simulink model "p2nftool_simulink"  (Simulink 7.7)
settings: Solver=ode45  StartTime=0.0  StopTime=10.0  RelTol=1e-3
libraries: neural x17
(part 1 of 3)
settings Model: Creator=Aditya  LastModifiedBy=Aditya

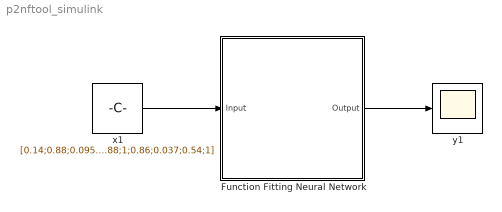
== system p2nftool_simulink ==
  Function Fitting Neural Network : Subsystem
      mask Description: Function Fitting Neural Network
      mask Display: e = 0.06;c1 = [120 150 230]/255;c2 = ([120 150 230]+0)/383;c3 = ([120 150 230]+128)/383;patch([0 1 1 0],[0 0 1 1],c1);patch([0 1 1 1-e 1-e 0+e],[0 0 1 1-e 0+e 0+e],c2);patch([0 0 1 1-e 0+e 0+e],[0 1 1 1-e 1-e 0+e],c3);plot([0 1 1 0 0],[0 0 1 1 0]);fprintf('NNET');port_label('input',1,' Input');port_label('output',1,'Output ');
  x1 : Constant  Value=[0.14;0.88;0.095;0.35;0.59;0.59;0.67;0.65;0.43;0.14;0.75;0.24;0.65;0.86;0.084;0.97;0.031;0.84;0.84;0.05;0.55;0.94;0.32;0.81;0.6;0.79;0.8;0.05;0.28;0.65;0.49;0.97;0.75;0.57;0.3;0.26;0.89;0.45;0.82;0.098;0.86;0.028;0.9;0.9;0.52;0.12;0.18;0.71;0.83;0.035;0.76;0.96;0.34;0.64;0.34;0.22;0.79;0.72;0.28;0.58;0.42;0.092;0.024;0.49;0.28;0.34;0.29;0.17;0.4;0.7;0.2;0.67;0.44;0.43;0.18;0.19;0.62;0.27;0.56;0.94;0.71;0.68;0.96;0.78;0.61;0.95;0.06;0.27;0.99;0.77;0.48;0.68;0.42;0.38;0.21;0.38;0.03;0.47;0.33;0.98;0.56;0.85;0.41;0.46;0.83;0.99;0.52;0.93;0.74;0.57;0.97;0.82;0.96;0.65;0.38;0.48;0.91;0.015;0.16;0.47;0.54;0.06;0.66;0.89;0.11;0.44;0.28;0.99;0.61;0.25;0.13;0.55;0.83;0.84;0.83;0.2;0.54;0.87;0.12;0.86;0.9;0.22;0.077;0.47;0.84;0.47;0.41;0.5;0.13;0.13;0.87;0.6;0.27;0.86;0.058;0.46;0.72;0.34;0.4;0.53;0.89;0.78;0.069;0.28;0.38;0.86;0.42;0.24;0.6;0.48;0.9;0.93;0.82;0.71;0.74;0.9;0.065;0.34;0.0043;0.83;0.51;0.37;0.23;0.53;0.29;0.068;0.085;0.068;0.41;0.12;0.44;0.9;0.35;0.12;0.57;0.88;0.35;0.042;0.14;0.077;0.74;0.46;0.67;0.7;0.57;0.63;0.88;0.66;0.88;0.47;0.14;0.068;0.71;0.31;0.67;0.65;0.53;0.72;0.5;0.49;0.5;0.94;0.39;0.12;0.24;0.68;0.84;0.97;0.22;0.76;0.58;0.4;0.51;0.5;0.65;0.74;0.3;0.09;0.83;0.39;0.78;0.18;0.11;0.91;0.88;1;0.86;0.037;0.54;1]  SampleTime=1
      mask Display: e = 0.06;c1 = [120 230 180]/255;c2 = ([120 230 180]+0)/(256+128);c3 = ([120 230 180]+128)/(256+128);patch([0 1 1 0],[0 0 1 1],c1);patch([0 1 1 1-e 1-e 0+e],[0 0 1 1-e 0+e 0+e],c2);patch([0 0 1 1-e 0+e 0+e],[0 1 1 1-e 1-e 0+e],c3);plot([0 1 1 0 0],[0 0 1 1 0]);disp('Constant');
  y1 : Scope
      settings: DataFormat=Array
      mask Display: e = 0.06;c1 = [120 230 180]/255;c2 = ([120 230 180]+0)/(256+128);c3 = ([120 230 180]+128)/(256+128);patch([0 1 1 0],[0 0 1 1],c1);patch([0 1 1 1-e 1-e 0+e],[0 0 1 1-e 0+e 0+e],c2);patch([0 0 1 1-e 0+e 0+e],[0 1 1 1-e 1-e 0+e],c3);plot([0 1 1 0 0],[0 0 1 1 0]);plot([0.15 0.85 0.85 0.15 0.15],[0.5 0.5 0.85 0.85 0.5]);
  wires:
  x1/1 -> Function Fitting Neural Network/1(Input)
  Function Fitting Neural Network/1(Output) -> y1/1

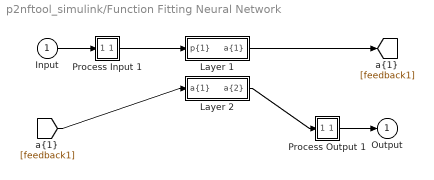
== system p2nftool_simulink/Function Fitting Neural Network ==
  Input : Inport  PortDimensions=250
      mask Display: e = 0.06;c1 = [120 230 180]/255;c2 = ([120 230 180]+0)/(256+128);c3 = ([120 230 180]+128)/(256+128);patch([0 1 1 0],[0 0 1 1],c1);patch([0 1 1 1-e 1-e 0+e],[0 0 1 1-e 0+e 0+e],c2);patch([0 0 1 1-e 0+e 0+e],[0 1 1 1-e 1-e 0+e],c3);plot([0 1 1 0 0],[0 0 1 1 0]);
  Layer 1 : Subsystem
      mask Display: e = 0.06;c1 = [120 150 230]/255;c2 = ([120 150 230]+0)/383;c3 = ([120 150 230]+128)/383;patch([0 1 1 0],[0 0 1 1],c1);patch([0 1 1 1-e 1-e 0+e],[0 0 1 1-e 0+e 0+e],c2);patch([0 0 1 1-e 0+e 0+e],[0 1 1 1-e 1-e 0+e],c3);plot([0 1 1 0 0],[0 0 1 1 0]);
  Layer 2 : Subsystem
      mask Display: e = 0.06;c1 = [120 150 230]/255;c2 = ([120 150 230]+0)/383;c3 = ([120 150 230]+128)/383;patch([0 1 1 0],[0 0 1 1],c1);patch([0 1 1 1-e 1-e 0+e],[0 0 1 1-e 0+e 0+e],c2);patch([0 0 1 1-e 0+e 0+e],[0 1 1 1-e 1-e 0+e],c3);plot([0 1 1 0 0],[0 0 1 1 0]);
  Process Input 1 : Subsystem
      mask Display: e = 0.06;c1 = [120 150 230]/255;c2 = ([120 150 230]+0)/383;c3 = ([120 150 230]+128)/383;patch([0 1 1 0],[0 0 1 1],c1);patch([0 1 1 1-e 1-e 0+e],[0 0 1 1-e 0+e 0+e],c2);patch([0 0 1 1-e 0+e 0+e],[0 1 1 1-e 1-e 0+e],c3);plot([0 1 1 0 0],[0 0 1 1 0]);
  Process Output 1 : Subsystem
      mask Display: e = 0.06;c1 = [120 150 230]/255;c2 = ([120 150 230]+0)/383;c3 = ([120 150 230]+128)/383;patch([0 1 1 0],[0 0 1 1],c1);patch([0 1 1 1-e 1-e 0+e],[0 0 1 1-e 0+e 0+e],c2);patch([0 0 1 1-e 0+e 0+e],[0 1 1 1-e 1-e 0+e],c3);plot([0 1 1 0 0],[0 0 1 1 0]);
  Output : Outport  InitialOutput=0
      mask Display: e = 0.06;c1 = [120 230 180]/255;c2 = ([120 230 180]+0)/(256+128);c3 = ([120 230 180]+128)/(256+128);patch([0 1 1 0],[0 0 1 1],c1);patch([0 1 1 1-e 1-e 0+e],[0 0 1 1-e 0+e 0+e],c2);patch([0 0 1 1-e 0+e 0+e],[0 1 1 1-e 1-e 0+e],c3);plot([0 1 1 0 0],[0 0 1 1 0]);
  wires:
  Input/1 -> Process Input 1/1(x)
  Process Output 1/1(y) -> Output/1
  Process Input 1/1(p) -> Layer 1/1("p{1}")
  Layer 1/1("a{1}") -> [feedback1]
  [feedback1] -> Layer 2/1("a{1} ")
  Layer 2/1("a{2}") -> Process Output 1/1(a)

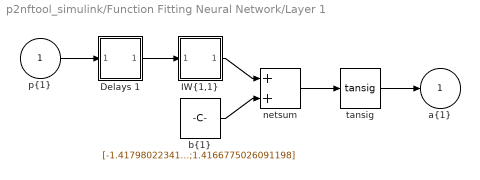
== system p2nftool_simulink/Function Fitting Neural Network/Layer 1 ==
  "p{1}" : Inport  PortDimensions=247
      mask Display: e = 0.06;c1 = [120 230 180]/255;c2 = ([120 230 180]+0)/(256+128);c3 = ([120 230 180]+128)/(256+128);patch([0 1 1 0],[0 0 1 1],c1);patch([0 1 1 1-e 1-e 0+e],[0 0 1 1-e 0+e 0+e],c2);patch([0 0 1 1-e 0+e 0+e],[0 1 1 1-e 1-e 0+e],c3);plot([0 1 1 0 0],[0 0 1 1 0]);
  Delays 1 : Subsystem
      mask Display: e = 0.06;c1 = [120 150 230]/255;c2 = ([120 150 230]+0)/383;c3 = ([120 150 230]+128)/383;patch([0 1 1 0],[0 0 1 1],c1);patch([0 1 1 1-e 1-e 0+e],[0 0 1 1-e 0+e 0+e],c2);patch([0 0 1 1-e 0+e 0+e],[0 1 1 1-e 1-e 0+e],c3);plot([0 1 1 0 0],[0 0 1 1 0]);disp('0');
  "IW{1,1}" : Subsystem
      mask Display: e = 0.06;c1 = [120 150 230]/255;c2 = ([120 150 230]+0)/383;c3 = ([120 150 230]+128)/383;patch([0 1 1 0],[0 0 1 1],c1);patch([0 1 1 1-e 1-e 0+e],[0 0 1 1-e 0+e 0+e],c2);patch([0 0 1 1-e 0+e 0+e],[0 1 1 1-e 1-e 0+e],c3);plot([0 1 1 0 0],[0 0 1 1 0]);disp('W');
  "b{1}" : Constant  Value=[-1.4179802234186696;-1.09460213536941;0.81514063966848649;-0.49229912761746891;-0.1249783039630278;-0.2000150392778885;-0.46243985430235329;0.78624382911976132;1.1056778923148194;1.4166775026091198]
      mask Display: e = 0.06;c1 = [120 150 230]/255;c2 = ([120 150 230]+0)/383;c3 = ([120 150 230]+128)/383;patch([0 1 1 0],[0 0 1 1],c1);patch([0 1 1 1-e 1-e 0+e],[0 0 1 1-e 0+e 0+e],c2);patch([0 0 1 1-e 0+e 0+e],[0 1 1 1-e 1-e 0+e],c3);plot([0 1 1 0 0],[0 0 1 1 0]);disp('b');
  netsum : Sum  Inputs=2  SaturateOnIntegerOverflow=on  InputSameDT=on  OutDataTypeStr=Inherit: Same as first input
      mask Display: e = 0.06;c1 = [120 150 230]/255;c2 = ([120 150 230]+0)/383;c3 = ([120 150 230]+128)/383;patch([0 1 1 0],[0 0 1 1],c1);patch([0 1 1 1-e 1-e 0+e],[0 0 1 1-e 0+e 0+e],c2);patch([0 0 1 1-e 0+e 0+e],[0 1 1 1-e 1-e 0+e],c3);plot([0 1 1 0 0],[0 0 1 1 0]);disp('+');
  tansig : neural/Transfer Functions/tansig  SystemSampleTime=-1
  "a{1}" : Outport  InitialOutput=[0;0;0;0;0;0;0;0;0;0]
      mask Display: e = 0.06;c1 = [120 230 180]/255;c2 = ([120 230 180]+0)/(256+128);c3 = ([120 230 180]+128)/(256+128);patch([0 1 1 0],[0 0 1 1],c1);patch([0 1 1 1-e 1-e 0+e],[0 0 1 1-e 0+e 0+e],c2);patch([0 0 1 1-e 0+e 0+e],[0 1 1 1-e 1-e 0+e],c3);plot([0 1 1 0 0],[0 0 1 1 0]);
  wires:
  "p{1}"/1 -> Delays 1/1("p{1}")
  Delays 1/1("pd{1,1}") -> "IW{1,1}"/1("pd{1,1}")
  "IW{1,1}"/1("iz{1,1}") -> netsum/1
  "b{1}"/1 -> netsum/2
  netsum/1 -> tansig/1
  tansig/1 -> "a{1}"/1

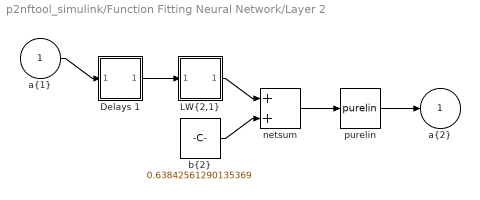
== system p2nftool_simulink/Function Fitting Neural Network/Layer 2 ==
  "a{1} " : Inport  PortDimensions=10
      mask Display: e = 0.06;c1 = [120 230 180]/255;c2 = ([120 230 180]+0)/(256+128);c3 = ([120 230 180]+128)/(256+128);patch([0 1 1 0],[0 0 1 1],c1);patch([0 1 1 1-e 1-e 0+e],[0 0 1 1-e 0+e 0+e],c2);patch([0 0 1 1-e 0+e 0+e],[0 1 1 1-e 1-e 0+e],c3);plot([0 1 1 0 0],[0 0 1 1 0]);
  Delays 1 : Subsystem
      mask Display: e = 0.06;c1 = [120 150 230]/255;c2 = ([120 150 230]+0)/383;c3 = ([120 150 230]+128)/383;patch([0 1 1 0],[0 0 1 1],c1);patch([0 1 1 1-e 1-e 0+e],[0 0 1 1-e 0+e 0+e],c2);patch([0 0 1 1-e 0+e 0+e],[0 1 1 1-e 1-e 0+e],c3);plot([0 1 1 0 0],[0 0 1 1 0]);disp('0');
  "LW{2,1}" : Subsystem
      mask Display: e = 0.06;c1 = [120 150 230]/255;c2 = ([120 150 230]+0)/383;c3 = ([120 150 230]+128)/383;patch([0 1 1 0],[0 0 1 1],c1);patch([0 1 1 1-e 1-e 0+e],[0 0 1 1-e 0+e 0+e],c2);patch([0 0 1 1-e 0+e 0+e],[0 1 1 1-e 1-e 0+e],c3);plot([0 1 1 0 0],[0 0 1 1 0]);disp('W');
  "b{2}" : Constant  Value=0.63842561290135369
      mask Display: e = 0.06;c1 = [120 150 230]/255;c2 = ([120 150 230]+0)/383;c3 = ([120 150 230]+128)/383;patch([0 1 1 0],[0 0 1 1],c1);patch([0 1 1 1-e 1-e 0+e],[0 0 1 1-e 0+e 0+e],c2);patch([0 0 1 1-e 0+e 0+e],[0 1 1 1-e 1-e 0+e],c3);plot([0 1 1 0 0],[0 0 1 1 0]);disp('b');
  netsum : Sum  Inputs=2  SaturateOnIntegerOverflow=on  InputSameDT=on  OutDataTypeStr=Inherit: Same as first input
      mask Display: e = 0.06;c1 = [120 150 230]/255;c2 = ([120 150 230]+0)/383;c3 = ([120 150 230]+128)/383;patch([0 1 1 0],[0 0 1 1],c1);patch([0 1 1 1-e 1-e 0+e],[0 0 1 1-e 0+e 0+e],c2);patch([0 0 1 1-e 0+e 0+e],[0 1 1 1-e 1-e 0+e],c3);plot([0 1 1 0 0],[0 0 1 1 0]);disp('+');
  purelin : neural/Transfer Functions/purelin  SystemSampleTime=-1
  "a{2}" : Outport  InitialOutput=0
      mask Display: e = 0.06;c1 = [120 230 180]/255;c2 = ([120 230 180]+0)/(256+128);c3 = ([120 230 180]+128)/(256+128);patch([0 1 1 0],[0 0 1 1],c1);patch([0 1 1 1-e 1-e 0+e],[0 0 1 1-e 0+e 0+e],c2);patch([0 0 1 1-e 0+e 0+e],[0 1 1 1-e 1-e 0+e],c3);plot([0 1 1 0 0],[0 0 1 1 0]);
  wires:
  "a{1} "/1 -> Delays 1/1("p{2}")
  Delays 1/1("pd{2,1}") -> "LW{2,1}"/1("ad{2,1}")
  "LW{2,1}"/1("lz{2,1}") -> netsum/1
  "b{2}"/1 -> netsum/2
  netsum/1 -> purelin/1
  purelin/1 -> "a{2}"/1

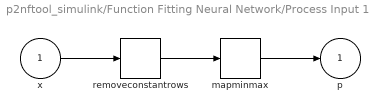
== system p2nftool_simulink/Function Fitting Neural Network/Process Input 1 ==
  x : Inport  PortDimensions=250
      mask Display: e = 0.06;c1 = [120 230 180]/255;c2 = ([120 230 180]+0)/(256+128);c3 = ([120 230 180]+128)/(256+128);patch([0 1 1 0],[0 0 1 1],c1);patch([0 1 1 1-e 1-e 0+e],[0 0 1 1-e 0+e 0+e],c2);patch([0 0 1 1-e 0+e 0+e],[0 1 1 1-e 1-e 0+e],c3);plot([0 1 1 0 0],[0 0 1 1 0]);
  mapminmax : neural/Processing Functions/mapminmax  SystemSampleTime=-1  xmin=[0.28314095380123011;0.0014657625514411762;1.1970013108086204e-053;0;3.1940747747761186e-136;1.0738088237835023e-008;0.057013843843753034;0.60598157151527954;0.97115785079355899;0.23505552379416098;0.0015659409791624098;1.7067224722511445e-053;0;8.0368942823302572e-061;4.5103371866006794e-009;0.04123819331054894;0.47948358616284426;0.88558703437196162;0.21511995153872421;0.0010808819751517852;2.8250692334704583e-046;2.4009309165522609e-100;2.9707490367076884e-027;9.6683230662484232e-007;0.022724192555573834;0.3373513142068964;0.94606039580726742;0.83381807044158585;0.21660287739295905;0.00088853633165548963;1.7009716611458678e-033;6.6780336252168211e-038;5.0696194701202741e-008;0.0036192264717555211;0.041362148979468445;0.30981136666700104;0.59801786498896425;0.79746531298425982;0.22315144476727924;0.0021495963375243315;8.1846160068553859e-025;2.8239914066742661e-017;0.0031408384351054031;0.042889224861903372;0.16276386773841925;0.40408038951216474;0.29066305341648024;0.76797757181136939;0.22877389647410262;0.0044456023366028895;5.600834653331497e-018;4.9394259822708177e-005;0.036840087959434539;0.17965949427207609;0.32363552339254342;0.45835299547326352;0.094130813464933724;0.75302798590493225;0.23743798347569076;0.0069561268877913604;6.4536346515668317e-010;0.008381002087497539;0.15708349906195013;0.30441724262311659;0.36780124819343157;0.2185871738005285;0.016765306036066845;0.74823061163344928;0.23947729804432752;0.010714512873083724;0.0010541317728196189;0.06157188394951027;0.28625369595068767;0.34844665670906477;0.28103818782833434;0.058728583468080235;0.0010252578856185749;0.74321854178214442;0.23689947649479201;0.018726205322830435;0.01403763154106394;0.22602305913201878;0.33322483120237623;0.33385806818767932;0.089161720319027582;0.0074641188499559637;4.9961895725867701e-014;0.73482943796744249;0.25372073679541962;0.029679290835118714;0.088110073989501325;0.30087532130095329;0.32980140896340393;0.16333410471453411;0.017268639637258193;2.1255584492753245e-005;3.393723053715393e-030;0.71603300903271727;0.28086288081641786;0.070765696337695222;0.25962114262595792;0.29530395857824981;0.29469508150713242;0.042775243878743575;0.0029717096345041856;2.9208044705741375e-016;6.5528308610418704e-056;0.69175545649373782;0.29982802434084543;0.20379814240139515;0.27454377432499888;0.27997276525054976;0.12616229517130753;0.0096590827511273004;1.3644328135045095e-006;2.142759325296534e-030;4.040485592604963e-142;0.66009817247140257;0.32061678791653081;0.2682547532557979;0.27174385900521508;0.20641766013384005;0.037985710799232193;0.0013807033350987767;1.3012635462117102e-015;5.4320946234375216e-057;1.7591464959013825e-240;0.6172769879756197;0.34847790967374298;0.26501955306395414;0.24801128848847065;0.060440114839899084;0.0055485797080829314;1.7011821839009803e-005;1.267314796215441e-026;4.0942538416128276e-118;0;0.55298588875176991;0.39441141595760654;0.24783748213069953;0.11231138884518392;0.010163982524210212;0.00014263917490065886;8.4779138948903329e-012;4.2832420373506433e-043;1.3914284431877022e-183;0;0.44408275342157744;0.45739136644383088;0.21373527300401277;0.030371879562093255;0.00095751904960731358;1.5885247614363501e-006;6.148043824133868e-020;7.3970467026419826e-081;1.4934597127927122e-257;0;0.26243962974132995;0.48079214069904203;0.26231548541471439;0.036602136267184941;0.00060628096867560799;1.2785305836116123e-008;1.1751484874139984e-028;1.1824443720758194e-113;1.5841675491774084e-254;0;0.090633848716506302;0.34771902491284706;0.38815621070205064;0.074059197286721362;0.003659510261993704;1.2345059166718358e-008;8.313897839456496e-019;4.7510923797345716e-037;4.5302986409558723e-159;0;0.010447510961658907;0.12022109545632396;0.43641885135063363;0.17835412356961261;0.023094869323530314;0.0036055987469813863;1.6562419958457672e-006;2.3336559312165858e-018;1.2249443391194443e-049;7.8777061358525906e-305;2.9236537014494795e-005;0.012406243347218964;0.14829252040733829;0.46412790611608706;0.26210222673708705 ...(+1093 chars)]  xmax=[0.54696499822519751;0.018097615199448878;1.1211625874404843e-008;5.6770535681185055e-031;3.0020232501492485e-023;0.0021391516298108959;0.14989077001407924;1;1;0.51285806504859077;0.012524359149825833;3.7565294910936581e-008;8.8658980841575836e-016;8.8232922508452755e-016;0.001431874497486966;0.11011541950728011;0.74534542491818523;1;0.48923990729976458;0.010269229460599905;0.00012832810780790373;2.2351799345579169e-007;1.1761696155131968e-007;0.0079013681222223249;0.17244731798578716;0.71244774902097929;1;1;0.48140245816606869;0.047806463657213097;0.0081972329787444211;0.00086126759741684059;0.00067631735814793108;0.054522031032458694;0.44327965809411135;0.92459203478062935;1;1;0.49019971138734014;0.17395100080588385;0.065005975793286361;0.01416422714286911;0.012751094148073646;0.20944713469156914;0.78827123663686649;0.87081878078898467;0.95513016761074909;1;0.51122174001432474;0.29403679313756742;0.18568212819115559;0.075803332242896079;0.078401394267904906;0.50135204144083989;0.9664167423402531;0.58456418046873104;0.91739553578710931;1;0.53971323573207386;0.29149662177536673;0.27410880384568065;0.1837507683046567;0.29524394301616924;0.84674198186133631;0.84210071990954583;0.42497663820874571;0.88784360430489151;1;0.57121324179208999;0.22637434602283085;0.28034774373112925;0.26868308271974917;0.59953438584907626;0.97047208655755235;0.50805015525697472;0.34234261762679447;0.87771026590275036;1;0.60074874094814346;0.1916976426070201;0.25414704427969675;0.44993057603357373;0.88913380145795928;0.78092906980325061;0.25708018546662409;0.30771110138826629;0.87022341791434699;1;0.617306656443951;0.19934536258060637;0.3230232905928398;0.68829336578133204;0.95490583236234927;0.43227229211606583;0.22921735464334314;0.29281982938187762;0.85988787364640351;1;0.60630227597781849;0.30945921967509815;0.57138434730137322;0.91429431990444288;0.71818200551782518;0.26394601892423619;0.21426386186227164;0.28369191206670286;0.84562505813256228;1;0.56823312027864892;0.44863329749984288;0.71906026058361971;0.92350828111072714;0.3747432970237301;0.22909478028122401;0.19935616204016754;0.27379410767962531;0.8266315756856335;1;0.51953034271202558;0.60295589781616798;0.91300857377332856;0.66280494491038633;0.22143189882557401;0.2026398062267977;0.1962579230845605;0.31999660638663485;0.80287348923773216;1;0.59296613606001092;0.68686554535086453;0.87309352639261761;0.38035071945566451;0.19048604266347183;0.17957438027237879;0.19276008856692992;0.37383438414826858;0.77561353621643292;1;0.66370203949103279;0.81071578487663132;0.63855594243678315;0.18363161767842476;0.16886869838772173;0.16759119141941323;0.22916253663769068;0.41022006167831676;0.75522032032662323;1;0.73729449658897717;0.7538058199151334;0.3771078802273462;0.15562663623401607;0.15415334753614637;0.16006433070656098;0.29132092095713402;0.43491866548201041;0.75875179823799987;1;0.77180671800562406;0.5668273239134819;0.17155060451941492;0.1329185837986466;0.14311963764645053;0.15322599053717373;0.37231070306965769;0.45173063997351182;0.75898683140048251;0.83129415315023303;0.78769388341964497;0.6903898422838507;0.44895919763123077;0.1310799125816258;0.13227596328915173;0.20184463272049286;0.4103151322505435;0.46903573008910326;0.75524943678441836;0.54304909791427902;0.78030741474702103;0.79441543065435416;0.71400559919879147;0.41985876969231978;0.12847278188546379;0.27306427097241653;0.42596678627353968;0.47506640461712185;0.74784590697831133;0.15994733323285074;0.51367456324893335;0.76588478994661346;0.79540230108298482;0.74664876613427333;0.39156046661972882;0.34114884070619123;0.45291405207552665;0.48456629233600629;0.73631043009063002;0.00022893929550700675;0.11306261647576715;0.42301243689598156;0.73475156560803945;0.78957771166163848;0.76512552649234056;0.38458568107385055;0.47257093304093056;0.47483300931247441;0.71685442986576109;1.3818041240619991e-008;0.00074138417223213555;0.065984006680153626;0.31244947587072502;0.6524693757289467;0.77720367695162929;0.77128579804533637 ...(+697 chars)]  ymin=-1  ymax=1
  removeconstantrows : neural/Processing Functions/removeconstantrows  SystemSampleTime=-1  inputSize=250  keep=[2 3 4 5 6 7 8 9 11 12 13 14 15 16 17 18 19 21 22 23 24 25 26 27 28 29 30 31 32 33 34 35 36 37 38 39 40 41 42 43 44 45 46 47 48 49 50 51 52 53 54 55 56 57 58 59 60 61 62 63 64 65 66 67 68 69 70 71 72 73 74 75 76 77 78 79 80 81 82 83 84 85 86 87 88 89 90 91 92 93 94 95 96 97 98 99 100 101 102 103 104 105 106 107 108 109 110 111 112 113 114 115 116 117 118 119 120 121 122 123 124 125 126 127 128 129 130 131 132 133 134 135 136 137 138 139 140 141 142 143 144 145 146 147 148 149 150 151 152 153 154 155 156 157 158 159 160 161 162 163 164 165 166 167 168 169 170 171 172 173 174 175 176 177 178 179 180 181 182 183 184 185 186 187 188 189 190 191 192 193 194 195 196 197 198 199 200 201 202 203 204 205 206 207 208 209 210 211 212 213 214 215 216 217 218 219 220 221 222 223 224 225 226 227 228 229 230 231 232 233 234 235 236 237 238 239 240 241 242 243 244 245 246 247 248 249 250]
  p : Outport  PortDimensions=247
      mask Display: e = 0.06;c1 = [120 230 180]/255;c2 = ([120 230 180]+0)/(256+128);c3 = ([120 230 180]+128)/(256+128);patch([0 1 1 0],[0 0 1 1],c1);patch([0 1 1 1-e 1-e 0+e],[0 0 1 1-e 0+e 0+e],c2);patch([0 0 1 1-e 0+e 0+e],[0 1 1 1-e 1-e 0+e],c3);plot([0 1 1 0 0],[0 0 1 1 0]);
  wires:
  x/1 -> removeconstantrows/1
  removeconstantrows/1 -> mapminmax/1
  mapminmax/1 -> p/1

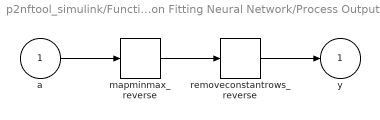
== system p2nftool_simulink/Function Fitting Neural Network/Process Output 1 ==
  a : Inport  PortDimensions=1
      mask Display: e = 0.06;c1 = [120 230 180]/255;c2 = ([120 230 180]+0)/(256+128);c3 = ([120 230 180]+128)/(256+128);patch([0 1 1 0],[0 0 1 1],c1);patch([0 1 1 1-e 1-e 0+e],[0 0 1 1-e 0+e 0+e],c2);patch([0 0 1 1-e 0+e 0+e],[0 1 1 1-e 1-e 0+e],c3);plot([0 1 1 0 0],[0 0 1 1 0]);
  mapminmax_reverse : neural/Processing Functions/mapminmax_reverse  SystemSampleTime=-1  xmin=-43.928813744888274  xmax=42.353350358455415  ymin=-1  ymax=1
  removeconstantrows_reverse : neural/Processing Functions/removeconstantrows_reverse  SystemSampleTime=-1  inputSize=1  constants=zeros(0,1)  rearrange=1
  y : Outport  PortDimensions=1
      mask Display: e = 0.06;c1 = [120 230 180]/255;c2 = ([120 230 180]+0)/(256+128);c3 = ([120 230 180]+128)/(256+128);patch([0 1 1 0],[0 0 1 1],c1);patch([0 1 1 1-e 1-e 0+e],[0 0 1 1-e 0+e 0+e],c2);patch([0 0 1 1-e 0+e 0+e],[0 1 1 1-e 1-e 0+e],c3);plot([0 1 1 0 0],[0 0 1 1 0]);
  wires:
  a/1 -> mapminmax_reverse/1
  mapminmax_reverse/1 -> removeconstantrows_reverse/1
  removeconstantrows_reverse/1 -> y/1

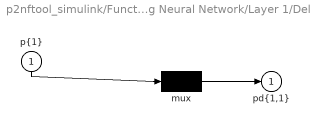
== system p2nftool_simulink/Function Fitting Neural Network/Layer 1/Delays 1 ==
  "p{1}" : Inport  PortDimensions=247
      mask Display: e = 0.06;c1 = [120 230 180]/255;c2 = ([120 230 180]+0)/(256+128);c3 = ([120 230 180]+128)/(256+128);patch([0 1 1 0],[0 0 1 1],c1);patch([0 1 1 1-e 1-e 0+e],[0 0 1 1-e 0+e 0+e],c2);patch([0 0 1 1-e 0+e 0+e],[0 1 1 1-e 1-e 0+e],c3);plot([0 1 1 0 0],[0 0 1 1 0]);
  mux : Mux  Inputs=1
      mask Display: e = 0.06;c1 = [120 150 230]/255;c2 = ([120 150 230]+0)/383;c3 = ([120 150 230]+128)/383;patch([0 1 1 0],[0 0 1 1],c1);patch([0 1 1 1-e 1-e 0+e],[0 0 1 1-e 0+e 0+e],c2);patch([0 0 1 1-e 0+e 0+e],[0 1 1 1-e 1-e 0+e],c3);plot([0 1 1 0 0],[0 0 1 1 0]);disp('Mux')
  "pd{1,1}" : Outport
      mask Display: e = 0.06;c1 = [120 230 180]/255;c2 = ([120 230 180]+0)/(256+128);c3 = ([120 230 180]+128)/(256+128);patch([0 1 1 0],[0 0 1 1],c1);patch([0 1 1 1-e 1-e 0+e],[0 0 1 1-e 0+e 0+e],c2);patch([0 0 1 1-e 0+e 0+e],[0 1 1 1-e 1-e 0+e],c3);plot([0 1 1 0 0],[0 0 1 1 0]);
  wires:
  "p{1}"/1 -> mux/1
  mux/1 -> "pd{1,1}"/1
